simulink model "Longitudinal_DynamicModel_ConstantSpeed"  (R2024b)
settings: Solver=VariableStepAuto  StartTime=0.0  StopTime=10.0  RelTol=1e-3
undefined symbols (not defined in the file or in its folder): car
libraries: simulink x1
settings Model: Creator=franc  LastModifiedBy=aless

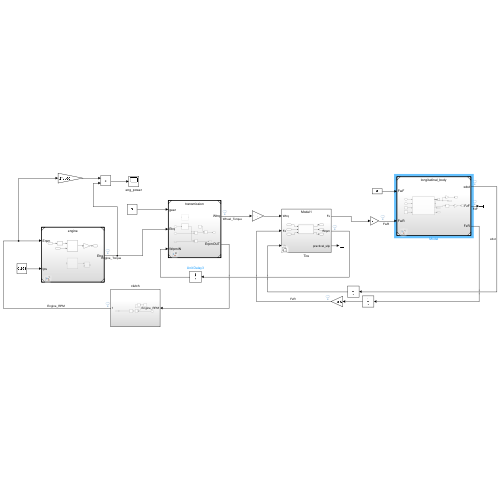
[thumbnail: Simulink's stored preview of the top-level diagram]
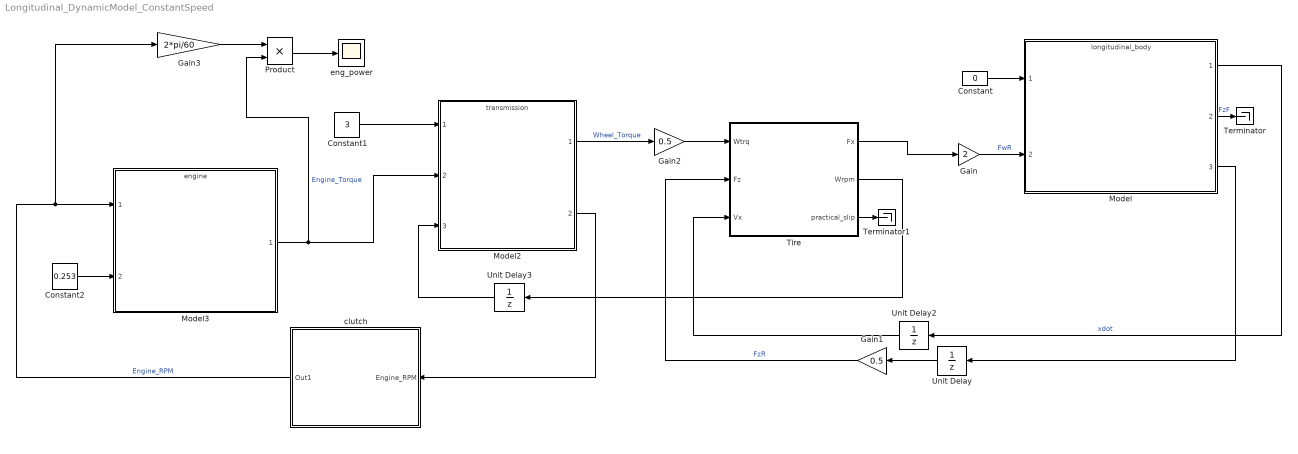
== system Longitudinal_DynamicModel_ConstantSpeed ==
  Constant : Constant  Value=0
  Constant1 : Constant  Value=3
  Constant2 : Constant  Value=0.253
  Gain : Gain  Gain=2
  Gain1 : Gain  Gain=0.5
  Gain2 : Gain  Gain=0.5
  Gain3 : Gain  Gain=2*pi/60
  Model : ModelReference  ModelNameDialog=longitudinal_body.slx  SimulationMode=Normal  ModelReferenceVersion=1.23
  Model2 : ModelReference  ModelNameDialog=transmission.slx  SimulationMode=Normal  ModelReferenceVersion=1.12
  Model3 : ModelReference  ModelNameDialog=engine.slx  SimulationMode=Normal  ModelReferenceVersion=1.18
  Product : Product
  Terminator : Terminator
  Terminator1 : Terminator
  Tire : Subsystem  Variant=on
  Unit Delay : UnitDelay  InitialCondition=car.initialconditions.FzR  SampleTime=-1  HasFrameUpgradeWarning=on
  Unit Delay2 : UnitDelay  InitialCondition=car.initialconditions.xdot  SampleTime=-1  HasFrameUpgradeWarning=on
  Unit Delay3 : UnitDelay  InitialCondition=car.initialconditions.Wrpm  SampleTime=-1  HasFrameUpgradeWarning=on
  clutch : Subsystem
  eng_power : Scope
  wires:
  Model3/1 -> Product/2, Model2/2  "Engine_Torque"
  Constant2/1 -> Model3/2
  Constant/1 -> Model/1
  Constant1/1 -> Model2/1
  Gain1/1 -> Tire/2(Fz)  "FzR"
  Unit Delay/1 -> Gain1/1
  Unit Delay2/1 -> Tire/3(Vx)
  Tire/2(Wrpm) -> Unit Delay3/1
  clutch/1(Out1) -> Gain3/1, Model3/1  "Engine_RPM"
  Model/1 -> Unit Delay2/1  "xdot"
  Gain2/1 -> Tire/1(Wtrq)
  Unit Delay3/1 -> Model2/3
  Tire/1(Fx) -> Gain/1
  Model/2 -> Terminator/1  "FzF"
  Gain/1 -> Model/2  "FwR"
  Tire/3(practical_slip) -> Terminator1/1
  Model2/1 -> Gain2/1  "Wheel_Torque"
  Model/3 -> Unit Delay/1
  Model2/2 -> clutch/1(Engine_RPM)
  Gain3/1 -> Product/1
  Product/1 -> eng_power/1

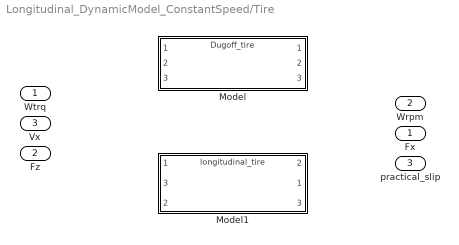
== system Longitudinal_DynamicModel_ConstantSpeed/Tire ==
  Wtrq : Inport
  Fz : Inport  Port=2
  Vx : Inport  Port=3
  Model : ModelReference  DisableCoverage=on  ModelNameDialog=Dugoff_tire.slx  SimulationMode=Normal  VariantControl=false  ModelReferenceVersion=2.16
  Model1 : ModelReference  ModelNameDialog=longitudinal_tire.slx  SimulationMode=Normal  VariantControl=true  ModelReferenceVersion=3.7
      settings: PortSchema="{\"entries\":[{\"content\":{\"sides\":[{\"content\":{\"connectorIds\":[\"In1\",\"In3\",\"In2\"]},\"type\":\"ConnectorPlacement.EquallySpacedRectSide\",\"uuid\":\"5eba1a74-bd07-49e9-ac91-356b950fcd72\"},{\"content\":{\"connectorIds\":[\"Out2\",\"Out1\",\"Out3\"],\"side\":\"RIGHT\"},\"type\":\"ConnectorPlacement.EquallySpacedRectSide\",\"uuid\":\"1040ce78-c535-419a-aa8f-ad6fbf19e979\"},{\"content\":{\"side\":\"TOP\"},\"type\":\"ConnectorPlacement.EquallySpacedRectSide\",\"uuid\":\"ba0f3e1f-76c3-4461-91cd-c7f47b575855\"}]},\"type\":\"ConnectorPlacement.EquallySpacedConnector\",\"uuid\":\"77c71335-a5e7-4e66-a78b-88921c7c7d22\"}],\"packageUris\":[\"http://schema.mathworks.com/mf0/Connector/R2020b\"],\"version\":\"1.0\"}"
  Fx : Outport
  Wrpm : Outport  Port=2
  practical_slip : Outport  Port=3

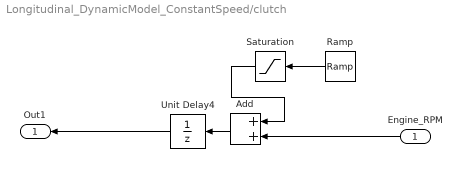
== system Longitudinal_DynamicModel_ConstantSpeed/clutch ==
  Engine_RPM : Inport
  Add : Sum
  Ramp : simulink/Sources/Ramp  slope=0  start=0  InitialOutput=0
  Saturation : Saturate  UpperLimit=car.initialconditions.EngineRPM  LowerLimit=0
  Unit Delay4 : UnitDelay  InitialCondition=car.initialconditions.EngineRPM  SampleTime=-1  HasFrameUpgradeWarning=on
  Out1 : Outport
  wires:
  Add/1 -> Unit Delay4/1
  Saturation/1 -> Add/1
  Ramp/1 -> Saturation/1
  Engine_RPM/1 -> Add/2
  Unit Delay4/1 -> Out1/1
